simulink model "Controller"  (R2015b)
settings: Solver=FixedStepAuto  StartTime=0.0  StopTime=inf  FixedStep=0.1  RelTol=1e-3
InitFcn:
  | robotics.ros.createSimulinkBus(gcs);
model workspace (MAT data in the model file):
  SL_ROS_VariableLengthArrays_MaxSizes.CommonInfo.ArrayTruncateAction = 'EmitWarning'
  SL_ROS_VariableLengthArrays_MaxSizes.MsgTypeMap = containers.Map
  SL_ROS_VariableLengthArrays_MaxSizes.MsgTypeMap.serialization.keys = {'std_msgs/Float32MultiArray', 'std_msgs/Float64MultiArray', 'std_msgs/Int64MultiArray', 'std_msgs/UInt16MultiArray'}
  SL_ROS_VariableLengthArrays_MaxSizes.MsgTypeMap.serialization.values{1}.PropertyName = 'Data'
  SL_ROS_VariableLengthArrays_MaxSizes.MsgTypeMap.serialization.values{1}.DataType = 'single'
  SL_ROS_VariableLengthArrays_MaxSizes.MsgTypeMap.serialization.values{1}.MaxLength = 10
  SL_ROS_VariableLengthArrays_MaxSizes.MsgTypeMap.serialization.values{2}.PropertyName = 'Data'
  SL_ROS_VariableLengthArrays_MaxSizes.MsgTypeMap.serialization.values{2}.DataType = 'double'
  SL_ROS_VariableLengthArrays_MaxSizes.MsgTypeMap.serialization.values{2}.MaxLength = 10
  SL_ROS_VariableLengthArrays_MaxSizes.MsgTypeMap.serialization.values{3}.PropertyName = 'Data'
  SL_ROS_VariableLengthArrays_MaxSizes.MsgTypeMap.serialization.values{3}.DataType = 'double'
  SL_ROS_VariableLengthArrays_MaxSizes.MsgTypeMap.serialization.values{3}.MaxLength = 10
  SL_ROS_VariableLengthArrays_MaxSizes.MsgTypeMap.serialization.values{4}.PropertyName = 'Data'
  SL_ROS_VariableLengthArrays_MaxSizes.MsgTypeMap.serialization.values{4}.DataType = 'uint16'
  SL_ROS_VariableLengthArrays_MaxSizes.MsgTypeMap.serialization.values{4}.MaxLength = 6
  SL_ROS_VariableLengthArrays_MaxSizes.MsgTypeMap.serialization.uniformity = 0
  SL_ROS_VariableLengthArrays_MaxSizes.MsgTypeMap.serialization.keyType = 'char'
  SL_ROS_VariableLengthArrays_MaxSizes.MsgTypeMap.serialization.valueType = 'any'
undefined symbols (not defined in the file or in its folder): DiscIntNeverNeededParam
libraries: robotlib x66, simulink x7, dspsrcs4 x6
(part 1 of 2)
settings Model: SimulationMode=accelerator  Creator=rasrack  LastModifiedBy=rasrack
settings OptimizationCC: OptimizeModelRefInitCode=on  LifeSpan=Inf  MaxStackSize=64
settings HardwareCC: ProdBitPerPointer=32  ProdLargestAtomicFloat=None  ProdIntDivRoundTo=Undefined  ProdEndianess=Unspecified  ProdWordSize=32  ProdHWDeviceType=Generic->Unspecified (assume 32-bit Generic)
settings ModelReferenceCC: EnableParallelModelReferenceBuilds=on
settings RTWCC: SystemTargetFile=ert.tlc  GenCodeOnly=on  TemplateMakefile=ert_default_tmf  Description=Embedded Coder  GenerateReport=on  Toolchain=Catkin  IncludeHyperlinkInReport=on  LaunchReport=on  TargetLang=C++  GenerateTraceInfo=on  GenerateTraceReport=on  GenerateTraceReportSl=on  GenerateTraceReportSf=on  GenerateTraceReportEml=on
settings CodeAppCC: ForceParamTrailComments=on  InternalIdentifier=Classic  ReqsInCode=on
settings ERTTargetCC: MultiInstanceERTCode=on  CodeInterfacePackaging=C++ class  SupportVariableSizeSignals=on  RootIOFormat=Structure reference

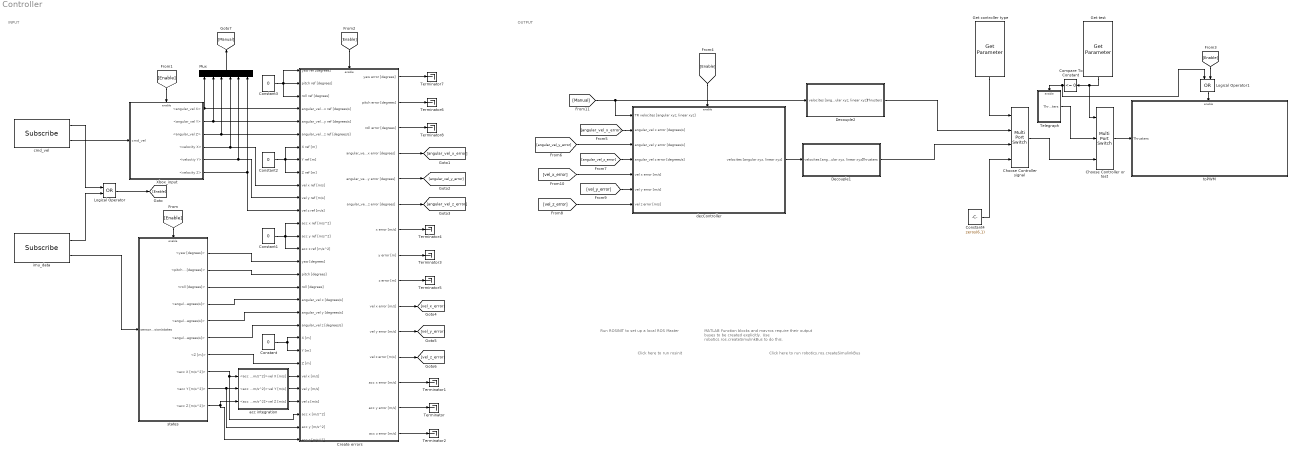
== system Controller ==
  note: INPUT
  note: OUTPUT
  note: Click here to run
      | robotics.ros.createSimulinkBus
  note: Run ROSINIT to set up a local ROS Master
  note: MATLAB Function blocks and mavros require their output buses to be created explicitly. Use robotics.ros.createSimulinkBus to do this.
  note: Click here to run
      | rosinit
  Choose Controller or test : MultiPortSwitch  DataPortOrder=Specify indices  DataPortIndices={0,1}
  Choose Controller signal : MultiPortSwitch  DataPortOrder=Specify indices  DataPortIndices={0,1,2}
  Compare To Constant : simulink/Logic and Bit Operations/Compare To Constant  relop=<=  const=0  OutDataTypeStr=boolean
  Constant{,1..3} (4 alike) : Constant  Value=0
  Constant4 : Constant  Value=zeros(6,1)
  Create errors : Subsystem
  Decouple1 : Subsystem
  Decouple2 : Subsystem
  Get controller type : robotlib/Get Parameter  SourceLibraryInfo=This block requires Robotics System Toolbox  ParameterSource=Select from ROS network  ParameterName=/matlab_controller/controller  ParameterType=int32  ParameterInitialValue=0  SampleTime=-1  ShowErrorCodeOutput=off  ModelName=Controller_without_ref  BlockId=ParamGet_Controller_without_ref_106
  Get test : robotlib/Get Parameter  SourceLibraryInfo=This block requires Robotics System Toolbox  ParameterSource=Specify your own  ParameterName=/matlab_controller/test  ParameterType=int32  ParameterInitialValue=1  SampleTime=-1  ShowErrorCodeOutput=off  ModelName=Controller_without_ref  BlockId=ParamGet_Controller_without_ref_823
  Logical Operator : Logic  Operator=OR  AllPortsSameDT=off  OutDataTypeStr=boolean
  Logical Operator1 : Logic  Operator=OR  AllPortsSameDT=off  OutDataTypeStr=boolean
  Mux : Mux  Inputs=6
  Telegraph : Subsystem
  Terminator{,1..8} (9 alike) : Terminator
  Xbox_input : Subsystem
  acc integration : Subsystem
  cmd_vel : robotlib/Subscribe  SourceLibraryInfo=This block requires Robotics System Toolbox  topicSource=Select from ROS network  topic=/cmd_vel  messageType=geometry_msgs/Twist  sampleTime=-1  messageQueueLength=10
  decController : Subsystem
  imu_data : robotlib/Subscribe  SourceLibraryInfo=This block requires Robotics System Toolbox  topicSource=Specify your own  topic=/sensor_fusion/states  messageType=std_msgs/Float64MultiArray  sampleTime=-1  messageQueueLength=10
  states : Subsystem  TreatAsAtomicUnit=on
  toPWM : Subsystem
  wires:
  cmd_vel/2 -> Xbox_input/1(cmd_vel)
  cmd_vel/1 -> Logical Operator/1
  imu_data/1 -> Logical Operator/2
  imu_data/2 -> states/1(sensor_fusion/states)
  Get controller type/1 -> Choose Controller signal/1
  Xbox_input/1(<angular_vel X>) -> Create errors/4(angular_vel x ref [degrees/s]), Mux/1
  Xbox_input/2(<angular_vel Y>) -> Mux/2, Create errors/5(angular_vel y ref [degrees/s])
  Xbox_input/3("<angular_vel Z> ") -> Mux/3, Create errors/6("angular_vel z ref [degrees/s] ")
  Xbox_input/4(<velocity X>) -> Mux/4, Create errors/10(vel x ref [m/s])
  Xbox_input/5(<veloctiy Y>) -> Mux/5, Create errors/11(vel y ref [m/s])
  Xbox_input/6(<velocity Z>) -> Create errors/12(vel z ref [m/s]), Mux/6
  states/1(<yaw [degrees]>) -> Create errors/16("yaw [degrees]  ")
  states/2(<pitch [degrees]>) -> Create errors/17(pitch [degrees])
  states/3(<roll [degrees]>) -> Create errors/18(roll [degrees])
  states/4(<angular_vel X [degrees/s]>) -> Create errors/19("angular_vel x [degrees/s]  ")
  states/5(<angular_vel Y [degrees/s]>) -> Create errors/20("angular_vel y [degrees/s] ")
  states/6(<angular_vel Z [degrees/s]>) -> Create errors/21(angular_vel z [degrees/s])
  Constant/1 -> Create errors/23(Y [m]), Create errors/22(X [m])
  acc integration/2(vel Y [m/s]) -> Create errors/26(vel y [m/s])
  acc integration/1("vel X [m/s] ") -> Create errors/25(vel x [m/s])
  acc integration/3(vel Z [m/s]) -> Create errors/27(vel z [m/s])
  states/8(<acc X [m/s^2]>) -> Create errors/28(acc x [m/s^2]), acc integration/1("<acc X [m/s^2]> ")
  states/9(<acc Y [m/s^2]>) -> Create errors/29(acc y [m/s^2]), acc integration/2(<acc Y [m/s^2]>)
  states/10(<acc Z [m/s^2]>) -> Create errors/30(acc z [m/s^2]), acc integration/3(<acc Z [m/s^2]>)
  Constant1/1 -> Create errors/15(acc z ref [m/s^2]), Create errors/13(acc x ref [m/s^2]), Create errors/14(acc y ref [m/s^2])
  Constant2/1 -> Create errors/9(Z ref [m]), Create errors/7(X ref [m]), Create errors/8(Y ref [m])
  Constant3/1 -> Create errors/1("yaw ref [degrees] "), Create errors/3(roll ref [degrees]), Create errors/2("pitch ref [degrees] ")
  Create errors/14(acc y error [m/s]) -> Terminator/1
  Create errors/13(acc x error [m/s]) -> Terminator1/1
  Create errors/15(acc z error [m/s]) -> Terminator2/1
  Create errors/8(y error [m]) -> Terminator3/1
  Create errors/7(x error [m/s]) -> Terminator4/1
  Create errors/9(z error [m]) -> Terminator5/1
  Create errors/2(pitch error [degrees]) -> Terminator6/1
  Create errors/1(yaw error [degrees]) -> Terminator7/1
  Create errors/3(roll error [degrees]) -> Terminator8/1
  Constant4/1 -> Choose Controller signal/4
  Logical Operator/1 -> [Enable]
  [Enable] -> states/Enable
  [Enable] -> Xbox_input/Enable
  [Enable] -> Create errors/Enable
  [Enable] -> decController/Enable
  Create errors/4(angular_vel x error [degrees]) -> [angular_vel_x_error]
  Create errors/5(angular_vel y error [degrees]) -> [angular_vel_y_error]
  Create errors/6(angular_vel z error [degrees]) -> [angular_vel_z_error]
  [angular_vel_x_error] -> decController/2("angular_vel x error [degrees/s] ")
  [angular_vel_y_error] -> decController/3(angular_vel y error [degrees/s])
  [angular_vel_z_error] -> decController/4(angular_vel z error [degrees/s])
  Create errors/10(vel x error [m/s]) -> [vel_x_error]
  Create errors/11(vel y error [m/s]) -> [vel_y_error]
  Create errors/12(vel z error [m/s]) -> [vel_z_error]
  [vel_z_error] -> decController/7("vel z error [m/s] ")
  [vel_y_error] -> decController/6("vel y error [m/s] ")
  [vel_x_error] -> decController/5("vel x error [m/s] ")
  Mux/1 -> [Manual]
  [Manual] -> Decouple2/1("velocites [angular xyz, linear xyz]    "), decController/1("TR velocites [angular xyz, linear xyz]  ")
  states/7(<Z [m]>) -> Create errors/24(Z [m])
  decController/1("velocites [angular xyz, linear xyz]") -> Decouple1/1("velocites [angular xyz, linear xyz]    ")
  Decouple1/1(Thrusters) -> Choose Controller signal/3
  Decouple2/1(Thrusters) -> Choose Controller signal/2
  Telegraph/1(Thrusters) -> Choose Controller or test/2
  Compare To Constant/1 -> Telegraph/Enable, Logical Operator1/1
  Choose Controller signal/1 -> Choose Controller or test/3
  [Enable] -> Logical Operator1/2
  Logical Operator1/1 -> toPWM/Enable
  Choose Controller or test/1 -> toPWM/1(Thrusters)
  Get test/1 -> Compare To Constant/1, Choose Controller or test/1

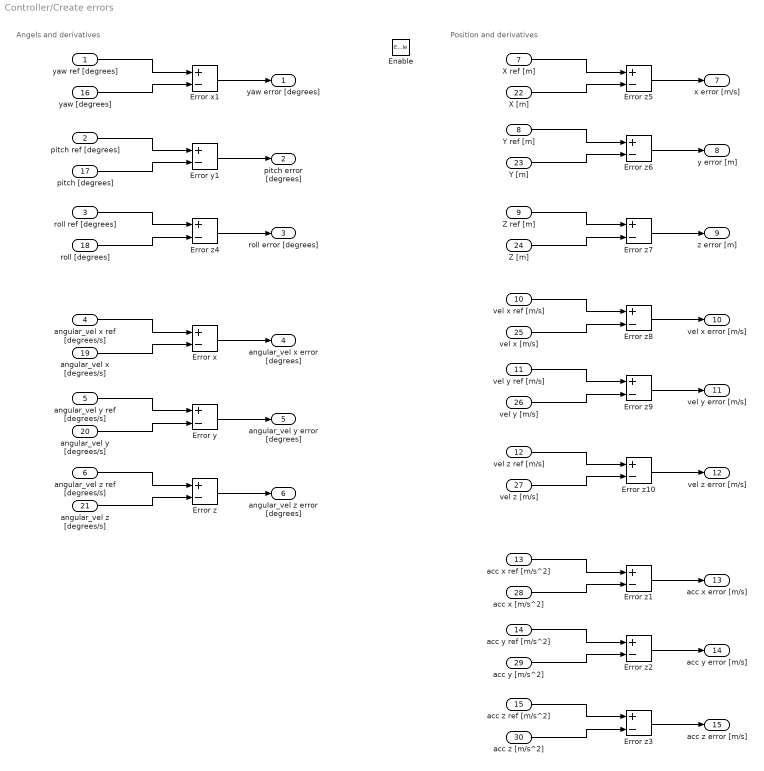
== system Controller/Create errors ==
  note: Position and derivatives
  note: Angels and derivatives
  "yaw ref [degrees] " : Inport
  "pitch ref [degrees] " : Inport  Port=2
  roll ref [degrees] : Inport  Port=3
  angular_vel x ref [degrees/s] : Inport  Port=4
  angular_vel y ref [degrees/s] : Inport  Port=5
  "angular_vel z ref [degrees/s] " : Inport  Port=6
  X ref [m] : Inport  Port=7
  Y ref [m] : Inport  Port=8
  Z ref [m] : Inport  Port=9
  vel x ref [m/s] : Inport  Port=10
  vel y ref [m/s] : Inport  Port=11
  vel z ref [m/s] : Inport  Port=12
  acc x ref [m/s^2] : Inport  Port=13
  acc y ref [m/s^2] : Inport  Port=14
  acc z ref [m/s^2] : Inport  Port=15
  "yaw [degrees]  " : Inport  Port=16
  pitch [degrees] : Inport  Port=17
  roll [degrees] : Inport  Port=18
  "angular_vel x [degrees/s]  " : Inport  Port=19
  "angular_vel y [degrees/s] " : Inport  Port=20
  angular_vel z [degrees/s] : Inport  Port=21
  X [m] : Inport  Port=22
  Y [m] : Inport  Port=23
  Z [m] : Inport  Port=24
  vel x [m/s] : Inport  Port=25
  vel y [m/s] : Inport  Port=26
  vel z [m/s] : Inport  Port=27
  acc x [m/s^2] : Inport  Port=28
  acc y [m/s^2] : Inport  Port=29
  acc z [m/s^2] : Inport  Port=30
  Enable : EnablePort
  Error x : Sum  Inputs=+-
  Error x1 : Sum  Inputs=+-
  Error y : Sum  Inputs=+-
  Error y1 : Sum  Inputs=+-
  Error z{,1..10} (11 alike) : Sum  Inputs=+-
  yaw error [degrees] : Outport
  pitch error [degrees] : Outport  Port=2
  roll error [degrees] : Outport  Port=3
  angular_vel x error [degrees] : Outport  Port=4
  angular_vel y error [degrees] : Outport  Port=5
  angular_vel z error [degrees] : Outport  Port=6
  x error [m/s] : Outport  Port=7
  y error [m] : Outport  Port=8
  z error [m] : Outport  Port=9
  vel x error [m/s] : Outport  Port=10
  vel y error [m/s] : Outport  Port=11
  vel z error [m/s] : Outport  Port=12
  acc x error [m/s] : Outport  Port=13
  acc y error [m/s] : Outport  Port=14
  acc z error [m/s] : Outport  Port=15
  wires:
  angular_vel x ref [degrees/s]/1 -> Error x/1
  "angular_vel x [degrees/s]  "/1 -> Error x/2
  Error x/1 -> angular_vel x error [degrees]/1
  angular_vel y ref [degrees/s]/1 -> Error y/1
  "angular_vel y [degrees/s] "/1 -> Error y/2
  Error y/1 -> angular_vel y error [degrees]/1
  "angular_vel z ref [degrees/s] "/1 -> Error z/1
  angular_vel z [degrees/s]/1 -> Error z/2
  Error z/1 -> angular_vel z error [degrees]/1
  acc x ref [m/s^2]/1 -> Error z1/1
  acc x [m/s^2]/1 -> Error z1/2
  Error z1/1 -> acc x error [m/s]/1
  acc y ref [m/s^2]/1 -> Error z2/1
  acc y [m/s^2]/1 -> Error z2/2
  Error z2/1 -> acc y error [m/s]/1
  acc z ref [m/s^2]/1 -> Error z3/1
  acc z [m/s^2]/1 -> Error z3/2
  Error z3/1 -> acc z error [m/s]/1
  "yaw ref [degrees] "/1 -> Error x1/1
  "yaw [degrees]  "/1 -> Error x1/2
  Error x1/1 -> yaw error [degrees]/1
  "pitch ref [degrees] "/1 -> Error y1/1
  pitch [degrees]/1 -> Error y1/2
  Error y1/1 -> pitch error [degrees]/1
  roll ref [degrees]/1 -> Error z4/1
  roll [degrees]/1 -> Error z4/2
  Error z4/1 -> roll error [degrees]/1
  X ref [m]/1 -> Error z5/1
  X [m]/1 -> Error z5/2
  Error z5/1 -> x error [m/s]/1
  Y ref [m]/1 -> Error z6/1
  Y [m]/1 -> Error z6/2
  Error z6/1 -> y error [m]/1
  Z ref [m]/1 -> Error z7/1
  Z [m]/1 -> Error z7/2
  Error z7/1 -> z error [m]/1
  vel x ref [m/s]/1 -> Error z8/1
  vel x [m/s]/1 -> Error z8/2
  Error z8/1 -> vel x error [m/s]/1
  vel y ref [m/s]/1 -> Error z9/1
  vel y [m/s]/1 -> Error z9/2
  Error z9/1 -> vel y error [m/s]/1
  vel z ref [m/s]/1 -> Error z10/1
  vel z [m/s]/1 -> Error z10/2
  Error z10/1 -> vel z error [m/s]/1

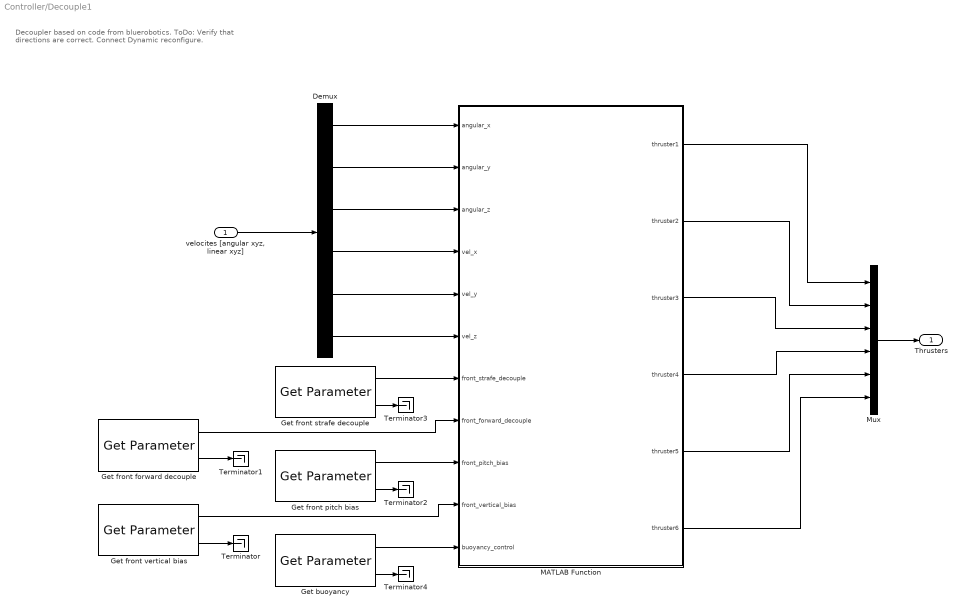
== system Controller/Decouple1 ==
  note: Decoupler based on code from bluerobotics.
      | ToDo:
      | Verify that directions are correct.
      | Connect Dynamic reconfigure.
  "velocites [angular xyz, linear xyz]    " : Inport
  Demux : Demux  Outputs=6
  Get buoyancy : robotlib/Get Parameter  SourceLibraryInfo=This block requires Robotics System Toolbox  ParameterSource=Select from ROS network  ParameterName=/matlab_controller/buoyancy_control  ParameterType=double  ParameterInitialValue=0.0  SampleTime=-1  ShowErrorCodeOutput=on  ModelName=Controller_without_ref  BlockId=ParamGet_Controller_without_ref_784
  Get front forward decouple : robotlib/Get Parameter  SourceLibraryInfo=This block requires Robotics System Toolbox  ParameterSource=Select from ROS network  ParameterName=/matlab_controller/front_forward_decouple  ParameterType=double  ParameterInitialValue=0.0  SampleTime=-1  ShowErrorCodeOutput=on  ModelName=Controller_without_ref  BlockId=ParamGet_Controller_without_ref_785
  Get front pitch bias : robotlib/Get Parameter  SourceLibraryInfo=This block requires Robotics System Toolbox  ParameterSource=Select from ROS network  ParameterName=/matlab_controller/front_pitch_bias  ParameterType=double  ParameterInitialValue=0.0  SampleTime=-1  ShowErrorCodeOutput=on  ModelName=Controller_without_ref  BlockId=ParamGet_Controller_without_ref_786
  Get front strafe decouple : robotlib/Get Parameter  SourceLibraryInfo=This block requires Robotics System Toolbox  ParameterSource=Select from ROS network  ParameterName=/matlab_controller/front_strafe_decouple  ParameterType=double  ParameterInitialValue=0.0  SampleTime=-1  ShowErrorCodeOutput=on  ModelName=Controller_without_ref  BlockId=ParamGet_Controller_without_ref_787
  Get front vertical bias : robotlib/Get Parameter  SourceLibraryInfo=This block requires Robotics System Toolbox  ParameterSource=Select from ROS network  ParameterName=/matlab_controller/front_vertical_bias  ParameterType=double  ParameterInitialValue=0.0  SampleTime=-1  ShowErrorCodeOutput=on  ModelName=Controller_without_ref  BlockId=ParamGet_Controller_without_ref_788
  MATLAB Function : MATLAB Function  TreatAsAtomicUnit=on
  Mux : Mux  Inputs=6
  Terminator{,1..4} (5 alike) : Terminator
  Thrusters : Outport
  wires:
  MATLAB Function/1(thruster1) -> Mux/1
  Get buoyancy/1 -> MATLAB Function/11(buoyancy_control)
  Get front vertical bias/1 -> MATLAB Function/10(front_vertical_bias)
  Get front pitch bias/1 -> MATLAB Function/9(front_pitch_bias)
  Get front forward decouple/1 -> MATLAB Function/8(front_forward_decouple)
  Get front strafe decouple/1 -> MATLAB Function/7(front_strafe_decouple)
  Demux/5 -> MATLAB Function/5(vel_y)
  Demux/6 -> MATLAB Function/6(vel_z)
  Demux/4 -> MATLAB Function/4(vel_x)
  Demux/3 -> MATLAB Function/3(angular_z)
  Demux/2 -> MATLAB Function/2(angular_y)
  Demux/1 -> MATLAB Function/1(angular_x)
  MATLAB Function/6(thruster6) -> Mux/6
  MATLAB Function/5(thruster5) -> Mux/5
  MATLAB Function/4(thruster4) -> Mux/4
  MATLAB Function/3(thruster3) -> Mux/3
  MATLAB Function/2(thruster2) -> Mux/2
  Get front vertical bias/2 -> Terminator/1
  Get front forward decouple/2 -> Terminator1/1
  Get front pitch bias/2 -> Terminator2/1
  Get front strafe decouple/2 -> Terminator3/1
  Get buoyancy/2 -> Terminator4/1
  "velocites [angular xyz, linear xyz]    "/1 -> Demux/1
  Mux/1 -> Thrusters/1

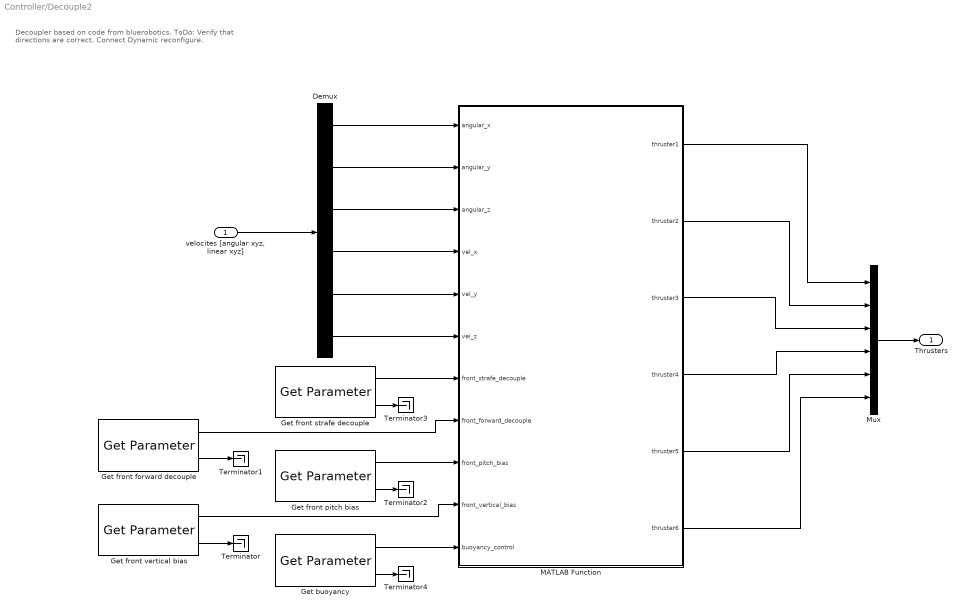
== system Controller/Decouple2 ==
  note: Decoupler based on code from bluerobotics.
      | ToDo:
      | Verify that directions are correct.
      | Connect Dynamic reconfigure.
  "velocites [angular xyz, linear xyz]    " : Inport
  Demux : Demux  Outputs=6
  Get buoyancy : robotlib/Get Parameter  SourceLibraryInfo=This block requires Robotics System Toolbox  ParameterSource=Select from ROS network  ParameterName=/matlab_controller/buoyancy_control  ParameterType=double  ParameterInitialValue=0.0  SampleTime=-1  ShowErrorCodeOutput=on  ModelName=Controller_without_ref  BlockId=ParamGet_Controller_without_ref_807
  Get front forward decouple : robotlib/Get Parameter  SourceLibraryInfo=This block requires Robotics System Toolbox  ParameterSource=Select from ROS network  ParameterName=/matlab_controller/front_forward_decouple  ParameterType=double  ParameterInitialValue=0.0  SampleTime=-1  ShowErrorCodeOutput=on  ModelName=Controller_without_ref  BlockId=ParamGet_Controller_without_ref_808
  Get front pitch bias : robotlib/Get Parameter  SourceLibraryInfo=This block requires Robotics System Toolbox  ParameterSource=Select from ROS network  ParameterName=/matlab_controller/front_pitch_bias  ParameterType=double  ParameterInitialValue=0.0  SampleTime=-1  ShowErrorCodeOutput=on  ModelName=Controller_without_ref  BlockId=ParamGet_Controller_without_ref_809
  Get front strafe decouple : robotlib/Get Parameter  SourceLibraryInfo=This block requires Robotics System Toolbox  ParameterSource=Select from ROS network  ParameterName=/matlab_controller/front_strafe_decouple  ParameterType=double  ParameterInitialValue=0.0  SampleTime=-1  ShowErrorCodeOutput=on  ModelName=Controller_without_ref  BlockId=ParamGet_Controller_without_ref_810
  Get front vertical bias : robotlib/Get Parameter  SourceLibraryInfo=This block requires Robotics System Toolbox  ParameterSource=Select from ROS network  ParameterName=/matlab_controller/front_vertical_bias  ParameterType=double  ParameterInitialValue=0.0  SampleTime=-1  ShowErrorCodeOutput=on  ModelName=Controller_without_ref  BlockId=ParamGet_Controller_without_ref_811
  MATLAB Function : MATLAB Function  TreatAsAtomicUnit=on
  Mux : Mux  Inputs=6
  Terminator{,1..4} (5 alike) : Terminator
  Thrusters : Outport
  wires:
  MATLAB Function/1(thruster1) -> Mux/1
  Get buoyancy/1 -> MATLAB Function/11(buoyancy_control)
  Get front vertical bias/1 -> MATLAB Function/10(front_vertical_bias)
  Get front pitch bias/1 -> MATLAB Function/9(front_pitch_bias)
  Get front forward decouple/1 -> MATLAB Function/8(front_forward_decouple)
  Get front strafe decouple/1 -> MATLAB Function/7(front_strafe_decouple)
  Demux/5 -> MATLAB Function/5(vel_y)
  Demux/6 -> MATLAB Function/6(vel_z)
  Demux/4 -> MATLAB Function/4(vel_x)
  Demux/3 -> MATLAB Function/3(angular_z)
  Demux/2 -> MATLAB Function/2(angular_y)
  Demux/1 -> MATLAB Function/1(angular_x)
  MATLAB Function/6(thruster6) -> Mux/6
  MATLAB Function/5(thruster5) -> Mux/5
  MATLAB Function/4(thruster4) -> Mux/4
  MATLAB Function/3(thruster3) -> Mux/3
  MATLAB Function/2(thruster2) -> Mux/2
  Get front vertical bias/2 -> Terminator/1
  Get front forward decouple/2 -> Terminator1/1
  Get front pitch bias/2 -> Terminator2/1
  Get front strafe decouple/2 -> Terminator3/1
  Get buoyancy/2 -> Terminator4/1
  "velocites [angular xyz, linear xyz]    "/1 -> Demux/1
  Mux/1 -> Thrusters/1

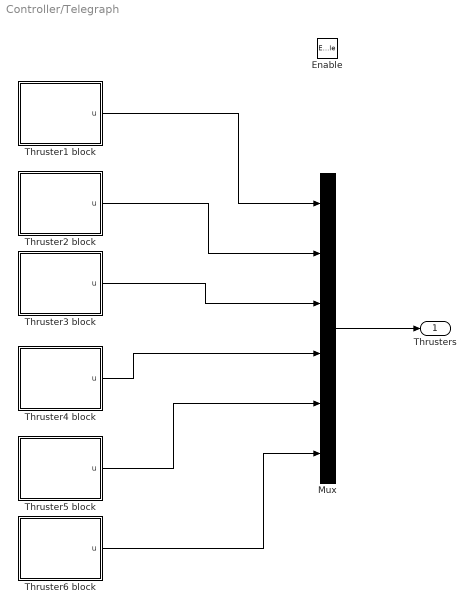
== system Controller/Telegraph ==
  Enable : EnablePort
  Mux : Mux  Inputs=6
  Thruster1 block : Subsystem
  Thruster2 block : Subsystem
  Thruster3 block : Subsystem
  Thruster4 block : Subsystem
  "Thruster5 block " : Subsystem
  Thruster6 block : Subsystem
  Thrusters : Outport
  wires:
  Mux/1 -> Thrusters/1
  Thruster1 block/1(u) -> Mux/1
  Thruster2 block/1(u) -> Mux/2
  Thruster3 block/1(u) -> Mux/3
  Thruster4 block/1(u) -> Mux/4
  "Thruster5 block "/1(u) -> Mux/5
  Thruster6 block/1(u) -> Mux/6

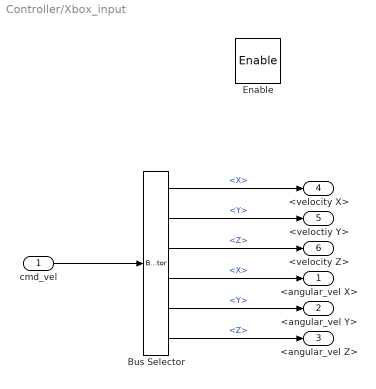
== system Controller/Xbox_input ==
  cmd_vel : Inport
  Enable : EnablePort
  Bus Selector : BusSelector  OutputSignals=Linear.X,Linear.Y,Linear.Z,Angular.X,Angular.Y,Angular.Z
  <angular_vel X> : Outport
  <angular_vel Y> : Outport  Port=2
  "<angular_vel Z> " : Outport  Port=3
  <velocity X> : Outport  Port=4
  <veloctiy Y> : Outport  Port=5
  <velocity Z> : Outport  Port=6
  wires:
  cmd_vel/1 -> Bus Selector/1
  Bus Selector/2 -> <veloctiy Y>/1  "<Y>"
  Bus Selector/1 -> <velocity X>/1  "<X>"
  Bus Selector/5 -> <angular_vel Y>/1  "<Y>"
  Bus Selector/3 -> <velocity Z>/1  "<Z>"
  Bus Selector/6 -> "<angular_vel Z> "/1  "<Z>"
  Bus Selector/4 -> <angular_vel X>/1  "<X>"

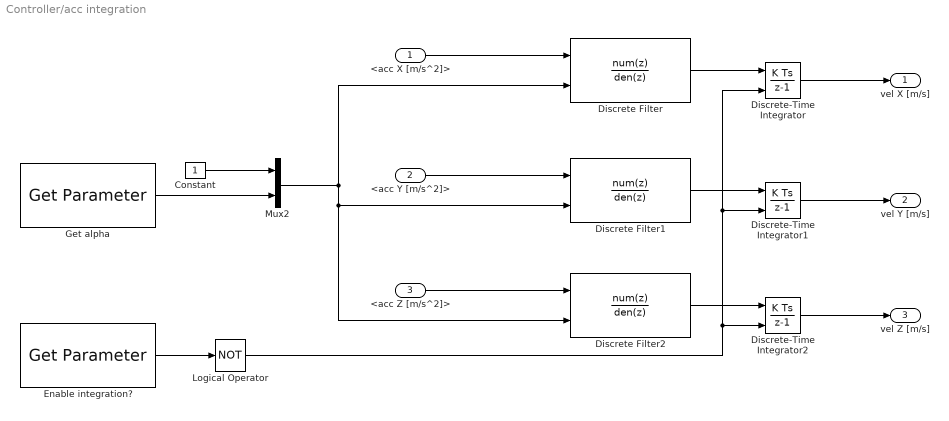
== system Controller/acc integration ==
  "<acc X [m/s^2]> " : Inport
  <acc Y [m/s^2]> : Inport  Port=2
  <acc Z [m/s^2]> : Inport  Port=3
  Constant : Constant
  Discrete Filter : DiscreteFilter  DenominatorSource=Input port  FilterStructure=Direct form I  a0EqualsOne=on
      settings: InputPortMap=u0,p3
  Discrete Filter1 : DiscreteFilter  DenominatorSource=Input port  FilterStructure=Direct form I  a0EqualsOne=on
      settings: InputPortMap=u0,p3
  Discrete Filter2 : DiscreteFilter  DenominatorSource=Input port  FilterStructure=Direct form I  a0EqualsOne=on
      settings: InputPortMap=u0,p3
  Discrete-Time Integrator : DiscreteIntegrator  ExternalReset=sampled level  InitialConditionSetting=State (most efficient)  SampleTime=-1  ICPrevOutput=DiscIntNeverNeededParam  ICPrevScaledInput=DiscIntNeverNeededParam
  Discrete-Time Integrator1 : DiscreteIntegrator  ExternalReset=sampled level  InitialConditionSetting=State (most efficient)  SampleTime=-1  ICPrevOutput=DiscIntNeverNeededParam  ICPrevScaledInput=DiscIntNeverNeededParam
  Discrete-Time Integrator2 : DiscreteIntegrator  ExternalReset=sampled level  InitialConditionSetting=State (most efficient)  SampleTime=-1  ICPrevOutput=DiscIntNeverNeededParam  ICPrevScaledInput=DiscIntNeverNeededParam
  Enable integration? : robotlib/Get Parameter  SourceLibraryInfo=This block requires Robotics System Toolbox  ParameterSource=Select from ROS network  ParameterName=/matlab_controller/enable_integration  ParameterType=boolean  ParameterInitialValue=0.0  SampleTime=-1  ShowErrorCodeOutput=off  ModelName=Controller_without_ref  BlockId=ParamGet_Controller_without_ref_686
  Get alpha : robotlib/Get Parameter  SourceLibraryInfo=This block requires Robotics System Toolbox  ParameterSource=Select from ROS network  ParameterName=/matlab_controller/alpha  ParameterType=double  ParameterInitialValue=0.0  SampleTime=-1  ShowErrorCodeOutput=off  ModelName=Controller_without_ref  BlockId=ParamGet_Controller_without_ref_687
  Logical Operator : Logic  Operator=NOT  AllPortsSameDT=off  OutDataTypeStr=boolean
  Mux2 : Mux  Inputs=2
  "vel X [m/s] " : Outport
  vel Y [m/s] : Outport  Port=2
  vel Z [m/s] : Outport  Port=3
  wires:
  Logical Operator/1 -> Discrete-Time Integrator2/2, Discrete-Time Integrator1/2, Discrete-Time Integrator/2
  Enable integration?/1 -> Logical Operator/1
  Constant/1 -> Mux2/1
  Get alpha/1 -> Mux2/2
  Mux2/1 -> Discrete Filter/2, Discrete Filter1/2, Discrete Filter2/2
  <acc Y [m/s^2]>/1 -> Discrete Filter1/1
  <acc Z [m/s^2]>/1 -> Discrete Filter2/1
  Discrete Filter2/1 -> Discrete-Time Integrator2/1
  Discrete Filter1/1 -> Discrete-Time Integrator1/1
  Discrete Filter/1 -> Discrete-Time Integrator/1
  "<acc X [m/s^2]> "/1 -> Discrete Filter/1
  Discrete-Time Integrator2/1 -> vel Z [m/s]/1
  Discrete-Time Integrator1/1 -> vel Y [m/s]/1
  Discrete-Time Integrator/1 -> "vel X [m/s] "/1

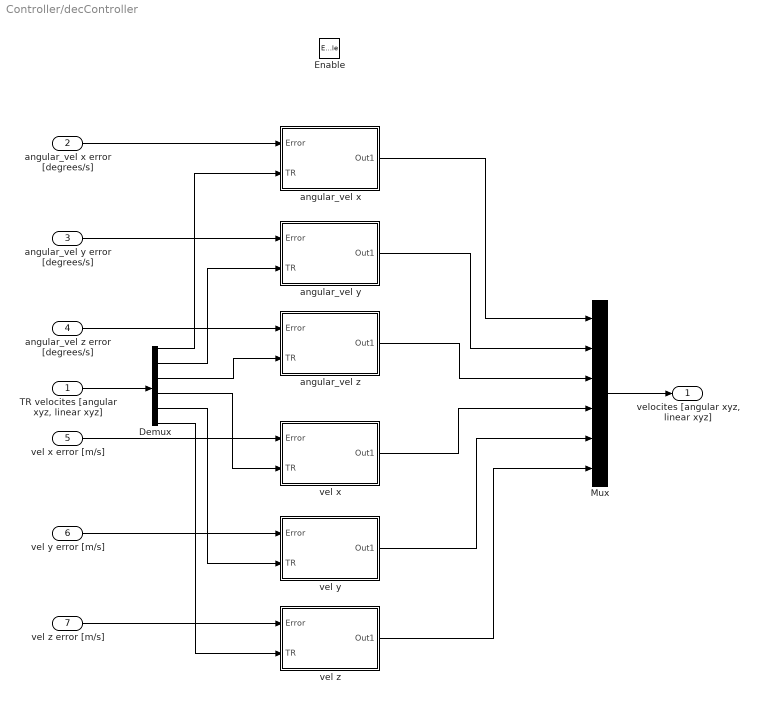
== system Controller/decController ==
  "TR velocites [angular xyz, linear xyz]  " : Inport
  "angular_vel x error [degrees/s] " : Inport  Port=2
  angular_vel y error [degrees/s] : Inport  Port=3
  angular_vel z error [degrees/s] : Inport  Port=4
  "vel x error [m/s] " : Inport  Port=5
  "vel y error [m/s] " : Inport  Port=6
  "vel z error [m/s] " : Inport  Port=7
  Enable : EnablePort  OutDataTypeStr=boolean
  Demux : Demux  Outputs=6
  Mux : Mux  Inputs=6
  angular_vel x : Subsystem
  angular_vel y : Subsystem
  angular_vel z : Subsystem
  vel x : Subsystem
  vel y : Subsystem
  vel z : Subsystem
  "velocites [angular xyz, linear xyz]" : Outport
  wires:
  "angular_vel x error [degrees/s] "/1 -> angular_vel x/1(Error)
  angular_vel y error [degrees/s]/1 -> angular_vel y/1(Error)
  angular_vel z error [degrees/s]/1 -> angular_vel z/1(Error)
  "vel x error [m/s] "/1 -> vel x/1(Error)
  "vel y error [m/s] "/1 -> vel y/1(Error)
  "vel z error [m/s] "/1 -> vel z/1(Error)
  vel z/1(Out1) -> Mux/6
  angular_vel x/1(Out1) -> Mux/1
  angular_vel y/1(Out1) -> Mux/2
  angular_vel z/1(Out1) -> Mux/3
  vel x/1(Out1) -> Mux/4
  vel y/1(Out1) -> Mux/5
  Mux/1 -> "velocites [angular xyz, linear xyz]"/1
  "TR velocites [angular xyz, linear xyz]  "/1 -> Demux/1
  Demux/1 -> angular_vel x/2(TR)
  Demux/2 -> angular_vel y/2(TR)
  Demux/3 -> angular_vel z/2(TR)
  Demux/4 -> vel x/2(TR)
  Demux/5 -> vel y/2(TR)
  Demux/6 -> vel z/2(TR)

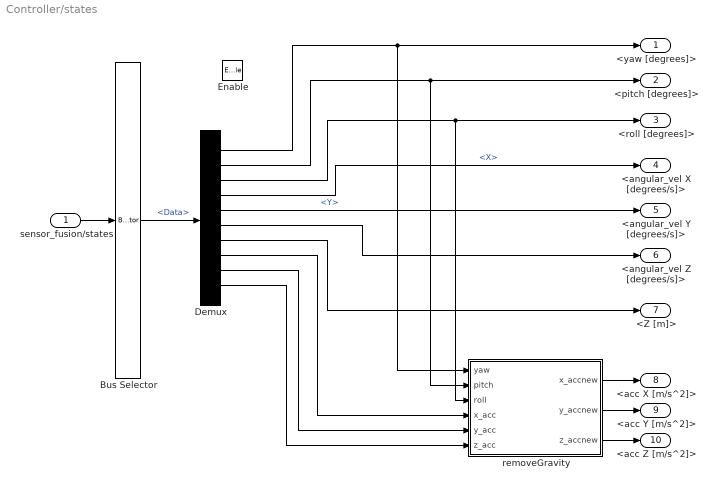
== system Controller/states ==
  sensor_fusion/states : Inport
  Enable : EnablePort
  Bus Selector : BusSelector  OutputSignals=Data
  Demux : Demux  Outputs=10
  removeGravity : MATLAB Function  TreatAsAtomicUnit=on
  <yaw [degrees]> : Outport
  <pitch [degrees]> : Outport  Port=2
  <roll [degrees]> : Outport  Port=3
  <angular_vel X [degrees/s]> : Outport  Port=4
  <angular_vel Y [degrees/s]> : Outport  Port=5
  <angular_vel Z [degrees/s]> : Outport  Port=6
  <Z [m]> : Outport  Port=7
  <acc X [m/s^2]> : Outport  Port=8
  <acc Y [m/s^2]> : Outport  Port=9
  <acc Z [m/s^2]> : Outport  Port=10
  wires:
  sensor_fusion/states/1 -> Bus Selector/1
  Demux/1 -> removeGravity/1(yaw), <yaw [degrees]>/1
  Demux/3 -> removeGravity/3(roll), <roll [degrees]>/1
  Demux/2 -> removeGravity/2(pitch), <pitch [degrees]>/1
  removeGravity/3(z_accnew) -> <acc Z [m/s^2]>/1
  removeGravity/2(y_accnew) -> <acc Y [m/s^2]>/1
  removeGravity/1(x_accnew) -> <acc X [m/s^2]>/1
  Demux/6 -> <angular_vel Z [degrees/s]>/1
  Bus Selector/1 -> Demux/1  "<Data>"
  Demux/4 -> <angular_vel X [degrees/s]>/1  "<X>"
  Demux/5 -> <angular_vel Y [degrees/s]>/1  "<Y>"
  Demux/7 -> <Z [m]>/1
  Demux/8 -> removeGravity/4(x_acc)
  Demux/9 -> removeGravity/5(y_acc)
  Demux/10 -> removeGravity/6(z_acc)

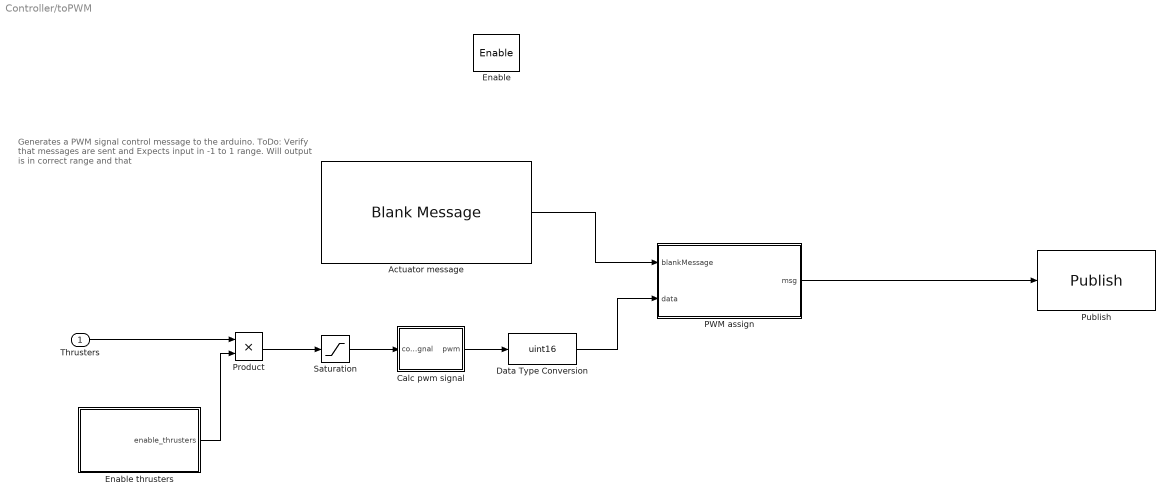
== system Controller/toPWM ==
  note: Generates a PWM signal control message to
      | the arduino.
      | ToDo:
      | Verify that messages are sent and
      | Expects input in -1 to 1 range.
      | Will output is in correct range and that
  Thrusters : Inport  PortDimensions=6
  Enable : EnablePort  OutDataTypeStr=boolean
  "Actuator message " : robotlib/Blank Message  SourceLibraryInfo=This block requires Robotics System Toolbox  messageType=std_msgs/UInt16MultiArray  SampleTime=-1
  Calc pwm signal : MATLAB Function  TreatAsAtomicUnit=on
  Data Type Conversion : DataTypeConversion  OutDataTypeStr=uint16
  "Enable thrusters " : Subsystem
  PWM assign : MATLAB Function  TreatAsAtomicUnit=on
  Product : Product
  Publish : robotlib/Publish  SourceLibraryInfo=This block requires Robotics System Toolbox  topicSource=Select from ROS network  topic=/rovio/thrusters  messageType=std_msgs/UInt16MultiArray  messageQueueLength=1
  Saturation : Saturate  UpperLimit=1  LowerLimit=-1
  wires:
  "Actuator message "/1 -> PWM assign/1(blankMessage)
  PWM assign/1(msg) -> Publish/1
  Saturation/1 -> Calc pwm signal/1(controlsignal)
  Calc pwm signal/1(pwm) -> Data Type Conversion/1
  Data Type Conversion/1 -> PWM assign/2(data)
  Thrusters/1 -> Product/1
  Product/1 -> Saturation/1
  "Enable thrusters "/1(enable_thrusters) -> Product/2

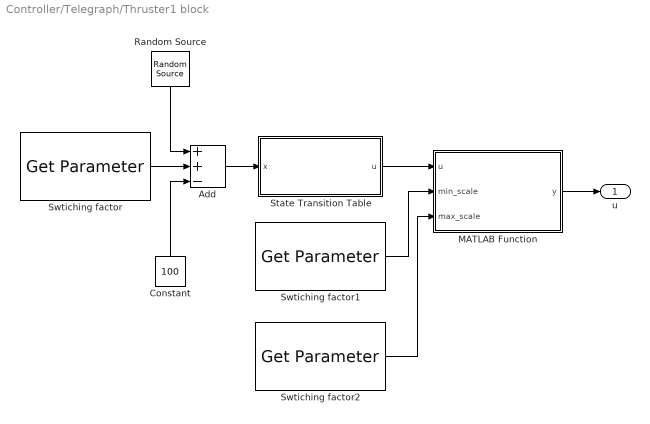
== system Controller/Telegraph/Thruster1 block ==
  Add : Sum  Inputs=++-
  Constant : Constant  Value=100
  MATLAB Function : MATLAB Function  TreatAsAtomicUnit=on
  Random Source : dspsrcs4/Random Source  SrcType=Uniform  NormMethod=Ziggurat  CltLength=12  MinVal=1  MaxVal=100  MeanVal=0  VarVal=1  RepMode=Not repeatable  rawSeed=1  IsInherit=on  SampMode=Discrete  SampTime=0.1  SampFrame=1  DataType=Double  OutComplex=Real  OutputFrames=off
  State Transition Table : State Transition Table  TreatAsAtomicUnit=on
  Swtiching factor : robotlib/Get Parameter  SourceLibraryInfo=This block requires Robotics System Toolbox  ParameterSource=Specify your own  ParameterName=/matlab_controller/switch_factor1  ParameterType=int32  ParameterInitialValue=0.0  SampleTime=-1  ShowErrorCodeOutput=off  ModelName=Controller_without_ref  BlockId=ParamGet_Controller_without_ref_714
  Swtiching factor1 : robotlib/Get Parameter  SourceLibraryInfo=This block requires Robotics System Toolbox  ParameterSource=Specify your own  ParameterName=/matlab_controller/min_scale1  ParameterType=double  ParameterInitialValue=1  SampleTime=-1  ShowErrorCodeOutput=off  ModelName=Controller_without_ref  BlockId=ParamGet_Controller_without_ref_715
  Swtiching factor2 : robotlib/Get Parameter  SourceLibraryInfo=This block requires Robotics System Toolbox  ParameterSource=Specify your own  ParameterName=/matlab_controller/max_scale1  ParameterType=double  ParameterInitialValue=1.0  SampleTime=-1  ShowErrorCodeOutput=off  ModelName=Controller_without_ref  BlockId=ParamGet_Controller_without_ref_716
  u : Outport
  wires:
  MATLAB Function/1(y) -> u/1
  Swtiching factor1/1 -> MATLAB Function/2(min_scale)
  State Transition Table/1(u) -> MATLAB Function/1(u)
  Swtiching factor2/1 -> MATLAB Function/3(max_scale)
  Add/1 -> State Transition Table/1(x)
  Swtiching factor/1 -> Add/2
  Random Source/1 -> Add/1
  Constant/1 -> Add/3

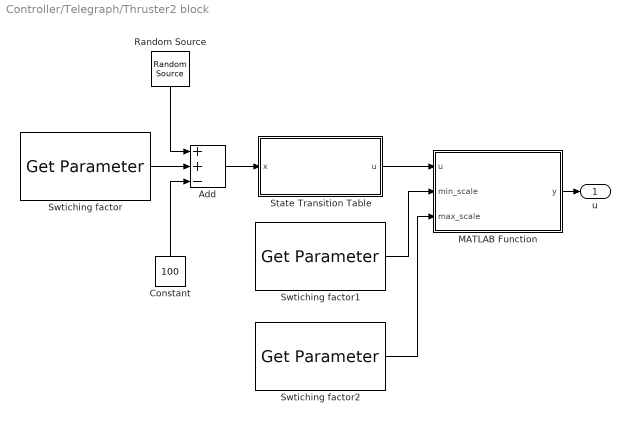
== system Controller/Telegraph/Thruster2 block ==
  Add : Sum  Inputs=++-
  Constant : Constant  Value=100
  MATLAB Function : MATLAB Function  TreatAsAtomicUnit=on
  Random Source : dspsrcs4/Random Source  SrcType=Uniform  NormMethod=Ziggurat  CltLength=12  MinVal=1  MaxVal=100  MeanVal=0  VarVal=1  RepMode=Not repeatable  rawSeed=1  IsInherit=on  SampMode=Discrete  SampTime=0.1  SampFrame=1  DataType=Double  OutComplex=Real  OutputFrames=off
  State Transition Table : State Transition Table  TreatAsAtomicUnit=on
  Swtiching factor : robotlib/Get Parameter  SourceLibraryInfo=This block requires Robotics System Toolbox  ParameterSource=Specify your own  ParameterName=/matlab_controller/switch_factor2  ParameterType=int32  ParameterInitialValue=0.0  SampleTime=-1  ShowErrorCodeOutput=off  ModelName=Controller_without_ref  BlockId=ParamGet_Controller_without_ref_724
  Swtiching factor1 : robotlib/Get Parameter  SourceLibraryInfo=This block requires Robotics System Toolbox  ParameterSource=Specify your own  ParameterName=/matlab_controller/min_scale2  ParameterType=double  ParameterInitialValue=1  SampleTime=-1  ShowErrorCodeOutput=off  ModelName=Controller_without_ref  BlockId=ParamGet_Controller_without_ref_725
  Swtiching factor2 : robotlib/Get Parameter  SourceLibraryInfo=This block requires Robotics System Toolbox  ParameterSource=Specify your own  ParameterName=/matlab_controller/max_scale2  ParameterType=double  ParameterInitialValue=1.0  SampleTime=-1  ShowErrorCodeOutput=off  ModelName=Controller_without_ref  BlockId=ParamGet_Controller_without_ref_726
  u : Outport
  wires:
  MATLAB Function/1(y) -> u/1
  Swtiching factor1/1 -> MATLAB Function/2(min_scale)
  State Transition Table/1(u) -> MATLAB Function/1(u)
  Swtiching factor2/1 -> MATLAB Function/3(max_scale)
  Add/1 -> State Transition Table/1(x)
  Swtiching factor/1 -> Add/2
  Random Source/1 -> Add/1
  Constant/1 -> Add/3

== system Controller/Telegraph/Thruster3 block ==
  Add : Sum  Inputs=++-
  Constant : Constant  Value=100
  MATLAB Function : MATLAB Function  TreatAsAtomicUnit=on
  Random Source : dspsrcs4/Random Source  SrcType=Uniform  NormMethod=Ziggurat  CltLength=12  MinVal=1  MaxVal=100  MeanVal=0  VarVal=1  RepMode=Not repeatable  rawSeed=1  IsInherit=on  SampMode=Discrete  SampTime=0.1  SampFrame=1  DataType=Double  OutComplex=Real  OutputFrames=off
  State Transition Table : State Transition Table  TreatAsAtomicUnit=on
  Swtiching factor : robotlib/Get Parameter  SourceLibraryInfo=This block requires Robotics System Toolbox  ParameterSource=Specify your own  ParameterName=/matlab_controller/switch_factor3  ParameterType=int32  ParameterInitialValue=0.0  SampleTime=-1  ShowErrorCodeOutput=off  ModelName=Controller_without_ref  BlockId=ParamGet_Controller_without_ref_734
  Swtiching factor1 : robotlib/Get Parameter  SourceLibraryInfo=This block requires Robotics System Toolbox  ParameterSource=Specify your own  ParameterName=/matlab_controller/min_scale3  ParameterType=double  ParameterInitialValue=1  SampleTime=-1  ShowErrorCodeOutput=off  ModelName=Controller_without_ref  BlockId=ParamGet_Controller_without_ref_735
  Swtiching factor2 : robotlib/Get Parameter  SourceLibraryInfo=This block requires Robotics System Toolbox  ParameterSource=Specify your own  ParameterName=/matlab_controller/max_scale3  ParameterType=double  ParameterInitialValue=1.0  SampleTime=-1  ShowErrorCodeOutput=off  ModelName=Controller_without_ref  BlockId=ParamGet_Controller_without_ref_736
  u : Outport
  wires:
  MATLAB Function/1(y) -> u/1
  Swtiching factor1/1 -> MATLAB Function/2(min_scale)
  State Transition Table/1(u) -> MATLAB Function/1(u)
  Swtiching factor2/1 -> MATLAB Function/3(max_scale)
  Add/1 -> State Transition Table/1(x)
  Swtiching factor/1 -> Add/2
  Random Source/1 -> Add/1
  Constant/1 -> Add/3

== system Controller/Telegraph/Thruster4 block ==
  Add : Sum  Inputs=++-
  Constant : Constant  Value=100
  MATLAB Function : MATLAB Function  TreatAsAtomicUnit=on
  Random Source : dspsrcs4/Random Source  SrcType=Uniform  NormMethod=Ziggurat  CltLength=12  MinVal=1  MaxVal=100  MeanVal=0  VarVal=1  RepMode=Not repeatable  rawSeed=1  IsInherit=on  SampMode=Discrete  SampTime=0.1  SampFrame=1  DataType=Double  OutComplex=Real  OutputFrames=off
  State Transition Table : State Transition Table  TreatAsAtomicUnit=on
  Swtiching factor : robotlib/Get Parameter  SourceLibraryInfo=This block requires Robotics System Toolbox  ParameterSource=Specify your own  ParameterName=/matlab_controller/switch_factor4  ParameterType=int32  ParameterInitialValue=0.0  SampleTime=-1  ShowErrorCodeOutput=off  ModelName=Controller_without_ref  BlockId=ParamGet_Controller_without_ref_744
  Swtiching factor1 : robotlib/Get Parameter  SourceLibraryInfo=This block requires Robotics System Toolbox  ParameterSource=Specify your own  ParameterName=/matlab_controller/min_scale4  ParameterType=double  ParameterInitialValue=1  SampleTime=-1  ShowErrorCodeOutput=off  ModelName=Controller_without_ref  BlockId=ParamGet_Controller_without_ref_745
  Swtiching factor2 : robotlib/Get Parameter  SourceLibraryInfo=This block requires Robotics System Toolbox  ParameterSource=Specify your own  ParameterName=/matlab_controller/max_scale4  ParameterType=double  ParameterInitialValue=1.0  SampleTime=-1  ShowErrorCodeOutput=off  ModelName=Controller_without_ref  BlockId=ParamGet_Controller_without_ref_746
  u : Outport
  wires:
  MATLAB Function/1(y) -> u/1
  Swtiching factor1/1 -> MATLAB Function/2(min_scale)
  State Transition Table/1(u) -> MATLAB Function/1(u)
  Swtiching factor2/1 -> MATLAB Function/3(max_scale)
  Add/1 -> State Transition Table/1(x)
  Swtiching factor/1 -> Add/2
  Random Source/1 -> Add/1
  Constant/1 -> Add/3

== system Controller/Telegraph/Thruster5 block  ==
  Add : Sum  Inputs=++-
  Constant : Constant  Value=100
  MATLAB Function : MATLAB Function  TreatAsAtomicUnit=on
  Random Source : dspsrcs4/Random Source  SrcType=Uniform  NormMethod=Ziggurat  CltLength=12  MinVal=1  MaxVal=100  MeanVal=0  VarVal=1  RepMode=Not repeatable  rawSeed=1  IsInherit=on  SampMode=Discrete  SampTime=0.1  SampFrame=1  DataType=Double  OutComplex=Real  OutputFrames=off
  State Transition Table : State Transition Table  TreatAsAtomicUnit=on
  Swtiching factor : robotlib/Get Parameter  SourceLibraryInfo=This block requires Robotics System Toolbox  ParameterSource=Specify your own  ParameterName=/matlab_controller/switch_factor5  ParameterType=int32  ParameterInitialValue=0.0  SampleTime=-1  ShowErrorCodeOutput=off  ModelName=Controller_without_ref  BlockId=ParamGet_Controller_without_ref_850
  Swtiching factor1 : robotlib/Get Parameter  SourceLibraryInfo=This block requires Robotics System Toolbox  ParameterSource=Specify your own  ParameterName=/matlab_controller/min_scale5  ParameterType=double  ParameterInitialValue=1  SampleTime=-1  ShowErrorCodeOutput=off  ModelName=Controller_without_ref  BlockId=ParamGet_Controller_without_ref_851
  Swtiching factor2 : robotlib/Get Parameter  SourceLibraryInfo=This block requires Robotics System Toolbox  ParameterSource=Specify your own  ParameterName=/matlab_controller/max_scale5  ParameterType=double  ParameterInitialValue=1.0  SampleTime=-1  ShowErrorCodeOutput=off  ModelName=Controller_without_ref  BlockId=ParamGet_Controller_without_ref_852
  u : Outport
  wires:
  MATLAB Function/1(y) -> u/1
  Swtiching factor1/1 -> MATLAB Function/2(min_scale)
  State Transition Table/1(u) -> MATLAB Function/1(u)
  Swtiching factor2/1 -> MATLAB Function/3(max_scale)
  Add/1 -> State Transition Table/1(x)
  Swtiching factor/1 -> Add/2
  Random Source/1 -> Add/1
  Constant/1 -> Add/3

== system Controller/Telegraph/Thruster6 block ==
  Add : Sum  Inputs=++-
  Constant : Constant  Value=100
  MATLAB Function : MATLAB Function  TreatAsAtomicUnit=on
  Random Source : dspsrcs4/Random Source  SrcType=Uniform  NormMethod=Ziggurat  CltLength=12  MinVal=1  MaxVal=100  MeanVal=0  VarVal=1  RepMode=Not repeatable  rawSeed=1  IsInherit=on  SampMode=Discrete  SampTime=0.1  SampFrame=1  DataType=Double  OutComplex=Real  OutputFrames=off
  State Transition Table : State Transition Table  TreatAsAtomicUnit=on
  Swtiching factor : robotlib/Get Parameter  SourceLibraryInfo=This block requires Robotics System Toolbox  ParameterSource=Specify your own  ParameterName=/matlab_controller/switch_factor6  ParameterType=int32  ParameterInitialValue=0.0  SampleTime=-1  ShowErrorCodeOutput=off  ModelName=Controller_without_ref  BlockId=ParamGet_Controller_without_ref_764
  Swtiching factor1 : robotlib/Get Parameter  SourceLibraryInfo=This block requires Robotics System Toolbox  ParameterSource=Specify your own  ParameterName=/matlab_controller/min_scale6  ParameterType=double  ParameterInitialValue=1  SampleTime=-1  ShowErrorCodeOutput=off  ModelName=Controller_without_ref  BlockId=ParamGet_Controller_without_ref_765
  Swtiching factor2 : robotlib/Get Parameter  SourceLibraryInfo=This block requires Robotics System Toolbox  ParameterSource=Specify your own  ParameterName=/matlab_controller/max_scale6  ParameterType=double  ParameterInitialValue=1.0  SampleTime=-1  ShowErrorCodeOutput=off  ModelName=Controller_without_ref  BlockId=ParamGet_Controller_without_ref_766
  u : Outport
  wires:
  MATLAB Function/1(y) -> u/1
  Swtiching factor1/1 -> MATLAB Function/2(min_scale)
  State Transition Table/1(u) -> MATLAB Function/1(u)
  Swtiching factor2/1 -> MATLAB Function/3(max_scale)
  Add/1 -> State Transition Table/1(x)
  Swtiching factor/1 -> Add/2
  Random Source/1 -> Add/1
  Constant/1 -> Add/3

== system Controller/decController/angular_vel x ==
  Error : Inport
  TR : Inport  Port=2
  PID Controller : simulink/Continuous/PID Controller  Controller=PID  TimeDomain=Discrete-time  SampleTime=-1  IntegratorMethod=Forward Euler  FilterMethod=Forward Euler  Form=Parallel  UseFilter=on  ControllerParametersSource=external  P=1  I=1  D=0  N=100  InitialConditionSource=internal  InitialConditionForIntegrator=0  InitialConditionForFilter=0  ExternalReset=none  LimitOutput=on  UpperSaturationLimit=1  LowerSaturationLimit=-1  LinearizeAsGain=on  AntiWindupMode=clamping  Kb=1  TrackingMode=on  Kt=1  SaturateOnIntegerOverflow=on  PParamMin=[]  PParamMax=[]  IParamMin=[]  IParamMax=[]  DParamMin=[]  DParamMax=[]  NParamMin=[]  NParamMax=[]  KbParamMin=[]  KbParamMax=[]  KtParamMin=[]  KtParamMax=[]  POutMin=[]  POutMax=[]  IOutMin=[]  IOutMax=[]  DOutMin=[]  DOutMax=[]  NOutMin=[]  NOutMax=[]  KbOutMin=[]  KbOutMax=[]  KtOutMin=[]  KtOutMax=[]  IntegratorOutMin=[]  IntegratorOutMax=[]  FilterOutMin=[]  FilterOutMax=[]  SumOutMin=[]  SumOutMax=[]  SumI1OutMin=[]  SumI1OutMax=[]  SumI2OutMin=[]  SumI2OutMax=[]  SumI3OutMin=[]  SumI3OutMax=[]  SumDOutMin=[]  SumDOutMax=[]  SaturationOutMin=[]  SaturationOutMax=[]  SaturationOutDataTypeStr=double  IntegratorContinuousStateAttributes=''  IntegratorStateMustResolveToSignalObject=off  IntegratorRTWStateStorageClass=Auto  FilterContinuousStateAttributes=''  FilterStateMustResolveToSignalObject=off  FilterRTWStateStorageClass=Auto  DifferentiatorICPrevScaledInput=0  DifferentiatorOutMin=[]  DifferentiatorOutMax=[]
  Retrive PID-Parameters : Subsystem
  Out1 : Outport
  wires:
  Retrive PID-Parameters/3(D) -> PID Controller/4
  Retrive PID-Parameters/2(I) -> PID Controller/3
  Retrive PID-Parameters/4(N) -> PID Controller/5
  Retrive PID-Parameters/1(P) -> PID Controller/2
  TR/1 -> PID Controller/6
  Error/1 -> PID Controller/1
  PID Controller/1 -> Out1/1

== system Controller/decController/angular_vel y ==
  Error : Inport
  TR : Inport  Port=2
  PID Controller : simulink/Continuous/PID Controller  Controller=PID  TimeDomain=Discrete-time  SampleTime=-1  IntegratorMethod=Forward Euler  FilterMethod=Forward Euler  Form=Parallel  UseFilter=on  ControllerParametersSource=external  P=1  I=1  D=0  N=100  InitialConditionSource=internal  InitialConditionForIntegrator=0  InitialConditionForFilter=0  ExternalReset=none  LimitOutput=on  UpperSaturationLimit=1  LowerSaturationLimit=-1  LinearizeAsGain=on  AntiWindupMode=clamping  Kb=1  TrackingMode=on  Kt=1  SaturateOnIntegerOverflow=on  PParamMin=[]  PParamMax=[]  IParamMin=[]  IParamMax=[]  DParamMin=[]  DParamMax=[]  NParamMin=[]  NParamMax=[]  KbParamMin=[]  KbParamMax=[]  KtParamMin=[]  KtParamMax=[]  POutMin=[]  POutMax=[]  IOutMin=[]  IOutMax=[]  DOutMin=[]  DOutMax=[]  NOutMin=[]  NOutMax=[]  KbOutMin=[]  KbOutMax=[]  KtOutMin=[]  KtOutMax=[]  IntegratorOutMin=[]  IntegratorOutMax=[]  FilterOutMin=[]  FilterOutMax=[]  SumOutMin=[]  SumOutMax=[]  SumI1OutMin=[]  SumI1OutMax=[]  SumI2OutMin=[]  SumI2OutMax=[]  SumI3OutMin=[]  SumI3OutMax=[]  SumDOutMin=[]  SumDOutMax=[]  SaturationOutMin=[]  SaturationOutMax=[]  IntegratorContinuousStateAttributes=''  IntegratorStateMustResolveToSignalObject=off  IntegratorRTWStateStorageClass=Auto  FilterContinuousStateAttributes=''  FilterStateMustResolveToSignalObject=off  FilterRTWStateStorageClass=Auto  DifferentiatorICPrevScaledInput=0  DifferentiatorOutMin=[]  DifferentiatorOutMax=[]
  Retrive PID-Parameters : Subsystem
  Out1 : Outport
  wires:
  Retrive PID-Parameters/3(D) -> PID Controller/4
  Retrive PID-Parameters/2(I) -> PID Controller/3
  Retrive PID-Parameters/4(N) -> PID Controller/5
  Retrive PID-Parameters/1(P) -> PID Controller/2
  TR/1 -> PID Controller/6
  Error/1 -> PID Controller/1
  PID Controller/1 -> Out1/1

== system Controller/decController/angular_vel z ==
  Error : Inport
  TR : Inport  Port=2
  PID Controller : simulink/Continuous/PID Controller  Controller=PID  TimeDomain=Discrete-time  SampleTime=-1  IntegratorMethod=Forward Euler  FilterMethod=Forward Euler  Form=Parallel  UseFilter=on  ControllerParametersSource=external  P=1  I=1  D=0  N=100  InitialConditionSource=internal  InitialConditionForIntegrator=0  InitialConditionForFilter=0  ExternalReset=none  LimitOutput=on  UpperSaturationLimit=1  LowerSaturationLimit=-1  LinearizeAsGain=on  AntiWindupMode=clamping  Kb=1  TrackingMode=on  Kt=1  SaturateOnIntegerOverflow=on  PParamMin=[]  PParamMax=[]  IParamMin=[]  IParamMax=[]  DParamMin=[]  DParamMax=[]  NParamMin=[]  NParamMax=[]  KbParamMin=[]  KbParamMax=[]  KtParamMin=[]  KtParamMax=[]  POutMin=[]  POutMax=[]  IOutMin=[]  IOutMax=[]  DOutMin=[]  DOutMax=[]  NOutMin=[]  NOutMax=[]  KbOutMin=[]  KbOutMax=[]  KtOutMin=[]  KtOutMax=[]  IntegratorOutMin=[]  IntegratorOutMax=[]  FilterOutMin=[]  FilterOutMax=[]  SumOutMin=[]  SumOutMax=[]  SumI1OutMin=[]  SumI1OutMax=[]  SumI2OutMin=[]  SumI2OutMax=[]  SumI3OutMin=[]  SumI3OutMax=[]  SumDOutMin=[]  SumDOutMax=[]  SaturationOutMin=[]  SaturationOutMax=[]  IntegratorContinuousStateAttributes=''  IntegratorStateMustResolveToSignalObject=off  IntegratorRTWStateStorageClass=Auto  FilterContinuousStateAttributes=''  FilterStateMustResolveToSignalObject=off  FilterRTWStateStorageClass=Auto  DifferentiatorICPrevScaledInput=0  DifferentiatorOutMin=[]  DifferentiatorOutMax=[]
  Retrive PID-Parameters : Subsystem
  Out1 : Outport
  wires:
  Retrive PID-Parameters/3(D) -> PID Controller/4
  Retrive PID-Parameters/2(I) -> PID Controller/3
  Retrive PID-Parameters/4(N) -> PID Controller/5
  Retrive PID-Parameters/1(P) -> PID Controller/2
  TR/1 -> PID Controller/6
  Error/1 -> PID Controller/1
  PID Controller/1 -> Out1/1

== system Controller/decController/vel x ==
  Error : Inport
  TR : Inport  Port=2
  PID Controller : simulink/Continuous/PID Controller  Controller=PID  TimeDomain=Discrete-time  SampleTime=-1  IntegratorMethod=Forward Euler  FilterMethod=Forward Euler  Form=Parallel  UseFilter=on  ControllerParametersSource=external  P=1  I=1  D=0  N=100  InitialConditionSource=internal  InitialConditionForIntegrator=0  InitialConditionForFilter=0  ExternalReset=none  LimitOutput=on  UpperSaturationLimit=1  LowerSaturationLimit=-1  LinearizeAsGain=on  AntiWindupMode=clamping  Kb=1  TrackingMode=on  Kt=1  SaturateOnIntegerOverflow=on  PParamMin=[]  PParamMax=[]  IParamMin=[]  IParamMax=[]  DParamMin=[]  DParamMax=[]  NParamMin=[]  NParamMax=[]  KbParamMin=[]  KbParamMax=[]  KtParamMin=[]  KtParamMax=[]  POutMin=[]  POutMax=[]  IOutMin=[]  IOutMax=[]  DOutMin=[]  DOutMax=[]  NOutMin=[]  NOutMax=[]  KbOutMin=[]  KbOutMax=[]  KtOutMin=[]  KtOutMax=[]  IntegratorOutMin=[]  IntegratorOutMax=[]  FilterOutMin=[]  FilterOutMax=[]  SumOutMin=[]  SumOutMax=[]  SumI1OutMin=[]  SumI1OutMax=[]  SumI2OutMin=[]  SumI2OutMax=[]  SumI3OutMin=[]  SumI3OutMax=[]  SumDOutMin=[]  SumDOutMax=[]  SaturationOutMin=[]  SaturationOutMax=[]  IntegratorContinuousStateAttributes=''  IntegratorStateMustResolveToSignalObject=off  IntegratorRTWStateStorageClass=Auto  FilterContinuousStateAttributes=''  FilterStateMustResolveToSignalObject=off  FilterRTWStateStorageClass=Auto  DifferentiatorICPrevScaledInput=0  DifferentiatorOutMin=[]  DifferentiatorOutMax=[]
  Retrive PID-Parameters : Subsystem
  Out1 : Outport
  wires:
  Retrive PID-Parameters/3(D) -> PID Controller/4
  Retrive PID-Parameters/2(I) -> PID Controller/3
  Retrive PID-Parameters/4(N) -> PID Controller/5
  Retrive PID-Parameters/1(P) -> PID Controller/2
  TR/1 -> PID Controller/6
  Error/1 -> PID Controller/1
  PID Controller/1 -> Out1/1

== system Controller/decController/vel y ==
  Error : Inport
  TR : Inport  Port=2
  PID Controller : simulink/Continuous/PID Controller  Controller=PID  TimeDomain=Discrete-time  SampleTime=-1  IntegratorMethod=Forward Euler  FilterMethod=Forward Euler  Form=Parallel  UseFilter=on  ControllerParametersSource=external  P=1  I=1  D=0  N=100  InitialConditionSource=internal  InitialConditionForIntegrator=0  InitialConditionForFilter=0  ExternalReset=none  LimitOutput=on  UpperSaturationLimit=1  LowerSaturationLimit=-1  LinearizeAsGain=on  AntiWindupMode=clamping  Kb=1  TrackingMode=on  Kt=1  SaturateOnIntegerOverflow=on  PParamMin=[]  PParamMax=[]  IParamMin=[]  IParamMax=[]  DParamMin=[]  DParamMax=[]  NParamMin=[]  NParamMax=[]  KbParamMin=[]  KbParamMax=[]  KtParamMin=[]  KtParamMax=[]  POutMin=[]  POutMax=[]  IOutMin=[]  IOutMax=[]  DOutMin=[]  DOutMax=[]  NOutMin=[]  NOutMax=[]  KbOutMin=[]  KbOutMax=[]  KtOutMin=[]  KtOutMax=[]  IntegratorOutMin=[]  IntegratorOutMax=[]  FilterOutMin=[]  FilterOutMax=[]  SumOutMin=[]  SumOutMax=[]  SumI1OutMin=[]  SumI1OutMax=[]  SumI2OutMin=[]  SumI2OutMax=[]  SumI3OutMin=[]  SumI3OutMax=[]  SumDOutMin=[]  SumDOutMax=[]  SaturationOutMin=[]  SaturationOutMax=[]  IntegratorContinuousStateAttributes=''  IntegratorStateMustResolveToSignalObject=off  IntegratorRTWStateStorageClass=Auto  FilterContinuousStateAttributes=''  FilterStateMustResolveToSignalObject=off  FilterRTWStateStorageClass=Auto  DifferentiatorICPrevScaledInput=0  DifferentiatorOutMin=[]  DifferentiatorOutMax=[]
  Retrive PID-Parameters : Subsystem
  Out1 : Outport
  wires:
  Retrive PID-Parameters/3(D) -> PID Controller/4
  Retrive PID-Parameters/2(I) -> PID Controller/3
  Retrive PID-Parameters/4(N) -> PID Controller/5
  Retrive PID-Parameters/1(P) -> PID Controller/2
  TR/1 -> PID Controller/6
  Error/1 -> PID Controller/1
  PID Controller/1 -> Out1/1

== system Controller/decController/vel z ==
  Error : Inport
  TR : Inport  Port=2
  PID Controller : simulink/Continuous/PID Controller  Controller=PID  TimeDomain=Discrete-time  SampleTime=-1  IntegratorMethod=Forward Euler  FilterMethod=Forward Euler  Form=Parallel  UseFilter=on  ControllerParametersSource=external  P=1  I=1  D=0  N=100  InitialConditionSource=internal  InitialConditionForIntegrator=0  InitialConditionForFilter=0  ExternalReset=none  LimitOutput=on  UpperSaturationLimit=1  LowerSaturationLimit=-1  LinearizeAsGain=on  AntiWindupMode=clamping  Kb=1  TrackingMode=on  Kt=1  SaturateOnIntegerOverflow=on  PParamMin=[]  PParamMax=[]  IParamMin=[]  IParamMax=[]  DParamMin=[]  DParamMax=[]  NParamMin=[]  NParamMax=[]  KbParamMin=[]  KbParamMax=[]  KtParamMin=[]  KtParamMax=[]  POutMin=[]  POutMax=[]  IOutMin=[]  IOutMax=[]  DOutMin=[]  DOutMax=[]  NOutMin=[]  NOutMax=[]  KbOutMin=[]  KbOutMax=[]  KtOutMin=[]  KtOutMax=[]  IntegratorOutMin=[]  IntegratorOutMax=[]  FilterOutMin=[]  FilterOutMax=[]  SumOutMin=[]  SumOutMax=[]  SumI1OutMin=[]  SumI1OutMax=[]  SumI2OutMin=[]  SumI2OutMax=[]  SumI3OutMin=[]  SumI3OutMax=[]  SumDOutMin=[]  SumDOutMax=[]  SaturationOutMin=[]  SaturationOutMax=[]  IntegratorContinuousStateAttributes=''  IntegratorStateMustResolveToSignalObject=off  IntegratorRTWStateStorageClass=Auto  FilterContinuousStateAttributes=''  FilterStateMustResolveToSignalObject=off  FilterRTWStateStorageClass=Auto  DifferentiatorICPrevScaledInput=0  DifferentiatorOutMin=[]  DifferentiatorOutMax=[]
  Retrive PID-Parameters : Subsystem
  Out1 : Outport
  wires:
  Retrive PID-Parameters/3(D) -> PID Controller/4
  Retrive PID-Parameters/2(I) -> PID Controller/3
  Retrive PID-Parameters/4(N) -> PID Controller/5
  Retrive PID-Parameters/1(P) -> PID Controller/2
  TR/1 -> PID Controller/6
  Error/1 -> PID Controller/1
  PID Controller/1 -> Out1/1
